simulink model "sprezyna_wahadlo_online"  (Simulink 7.5)
settings: Solver=ode45  StartTime=0.0  StopTime=100  RelTol=1e-3
settings Model: Creator=psoltysiak  LastModifiedBy=Soltys
settings DebuggingCC: StrictBusMsg=Warning

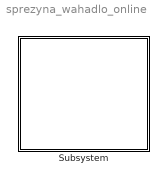
== system sprezyna_wahadlo_online ==
  Subsystem : Subsystem  mask{mk=5, mw=1, l=1, g=9.81, c=1, k1=0, k2=0, t0=0.01, phi0=45, z0=0.07}
      mask prompts: mk "MASA KLOCKA"; mw "masa wahadla"; l "dlugosc wahadla"; g "przyspieszenie"; c "stala sprezyny"; k1 "wspolczynnik oporu klocka"; k2 "wspolczynnik ooru klocka"; t0 "czas odswiezania"; phi0 "wychylenie wach poczatkowe"; z0 "wychylenie bloczka poczatkowe"

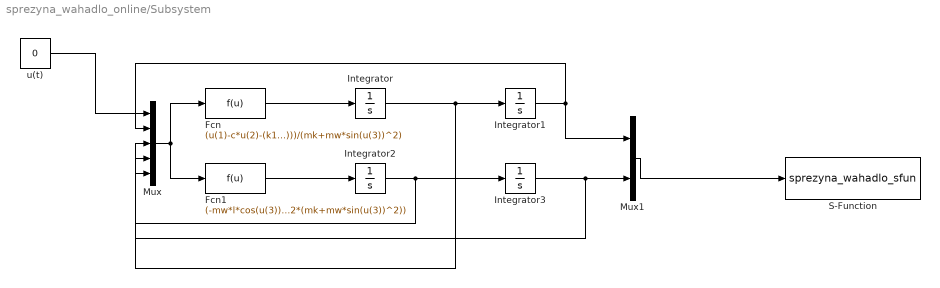
== system sprezyna_wahadlo_online/Subsystem ==
  Fcn : Fcn  Expr=(u(1)-c*u(2)-(k1+k2*sin(u(3))^2)*u(4)+mw*sin(u(3))*(l*u(5)^2+g*cos(u(3))))/(mk+mw*sin(u(3))^2)
  Fcn1 : Fcn  Expr=(-mw*l*cos(u(3))*(u(1))+mw*l*cos(u(3))*c*u(2)+l*cos(u(3))*(mw*k1-mk*k2)*u(4)-k2*l^2*(mk+mw*sin(u(3))^2)*u(5)-(mk+mw)*mw*g*l*sin(u(3))-mw^2*l^2*sin(u(3))*cos(u(3))*u(5)^2)/(mw*l^2*(mk+mw*sin(u(3))^2))
  Integrator : Integrator
  Integrator1 : Integrator  InitialCondition=z0
  Integrator2 : Integrator
  Integrator3 : Integrator  InitialCondition=phi0*pi/180
  Mux : Mux  Inputs=5
  Mux1 : Mux  Inputs=2
  S-Function : S-Function  FunctionName=sprezyna_wahadlo_sfun  Parameters=mk,mw,l,g,c,k1,k2,phi0,z0,t0  EnableBusSupport=off
  u(t) : Constant  Value=0  OutDataType=fixdt(1, 16)  OutScaling=2^0
  wires:
  Fcn/1 -> Integrator/1
  Integrator/1 -> Integrator1/1, Mux/4
  Fcn1/1 -> Integrator2/1
  Integrator2/1 -> Integrator3/1, Mux/5
  Integrator1/1 -> Mux/2, Mux1/1
  Integrator3/1 -> Mux/3, Mux1/2
  Mux/1 -> Fcn/1, Fcn1/1
  u(t)/1 -> Mux/1
  Mux1/1 -> S-Function/1
